simulink model "model_2"  (R2022a)
settings: Solver=FixedStepAuto  StartTime=0.0  StopTime=20  FixedStep=0.0001  RelTol=1e-3
libraries: cstblocks x2
settings Model: Creator=Family  LastModifiedBy=Family

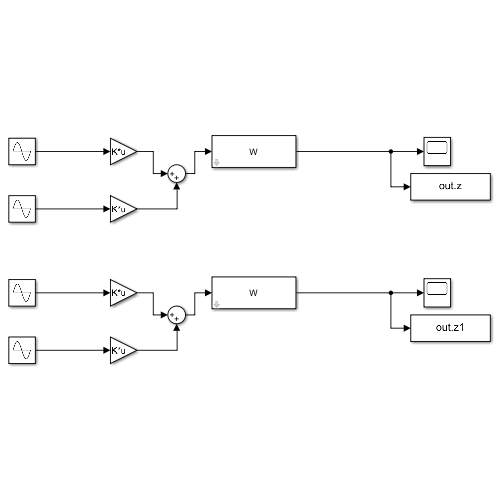
[thumbnail: Simulink's stored preview of the top-level diagram]
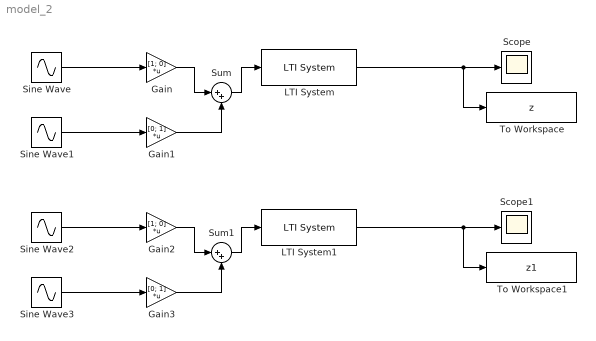
== system model_2 ==
  Gain : Gain  Gain=[1; 0]  Multiplication=Matrix(K*u)
  Gain1 : Gain  Gain=[0; 1]  Multiplication=Matrix(K*u)
  Gain2 : Gain  Gain=[1; 0]  Multiplication=Matrix(K*u)
  Gain3 : Gain  Gain=[0; 1]  Multiplication=Matrix(K*u)
  LTI System : cstblocks/LTI System  sys=W  IC=[]
  LTI System1 : cstblocks/LTI System  sys=W  IC=[]
  Scope : Scope
  Scope1 : Scope
  Sine Wave : Sin  Amplitude=2  Frequency=0.9  Phase=pi/4  SampleTime=0
  Sine Wave1 : Sin  Amplitude=3  Frequency=0.9  Phase=pi/2  SampleTime=0
  Sine Wave2 : Sin  Amplitude=2  Frequency=9  Phase=pi/4  SampleTime=0
  Sine Wave3 : Sin  Amplitude=3  Frequency=9  Phase=pi/2  SampleTime=0
  Sum : Sum  Inputs=|++
  Sum1 : Sum  Inputs=|++
  To Workspace : ToWorkspace  VariableName=z  SaveFormat=Timeseries  SampleTime=-1
  To Workspace1 : ToWorkspace  VariableName=z1  SaveFormat=Timeseries  SampleTime=-1
  wires:
  Sine Wave1/1 -> Gain1/1
  Gain/1 -> Sum/1
  Sine Wave/1 -> Gain/1
  Sum/1 -> LTI System/1
  LTI System/1 -> To Workspace/1, Scope/1
  Gain1/1 -> Sum/2
  LTI System1/1 -> To Workspace1/1, Scope1/1
  Gain3/1 -> Sum1/2
  Sine Wave2/1 -> Gain2/1
  Gain2/1 -> Sum1/1
  Sine Wave3/1 -> Gain3/1
  Sum1/1 -> LTI System1/1
